simulink model "VaRedoxFlowBattery"  (R2025b)
settings: Solver=daessc  StartTime=0.0  StopTime=217080  FixedStep=1  MaxStep=1  RelTol=1e-3
libraries: fl_lib x4, nesl_utility x2, energyStorage_lib x1
settings Model: Creator=The MathWorks, Inc.  LastModifiedBy=skota
settings DataIOCC: ReturnWorkspaceOutputs=off
settings RTWCC: GPUComputeCapability=3.5
settings SimscapeCC: SimscapeLogType=all  SimscapeLogName=simlog_vrfbResults  SimscapeLogLimitData=off

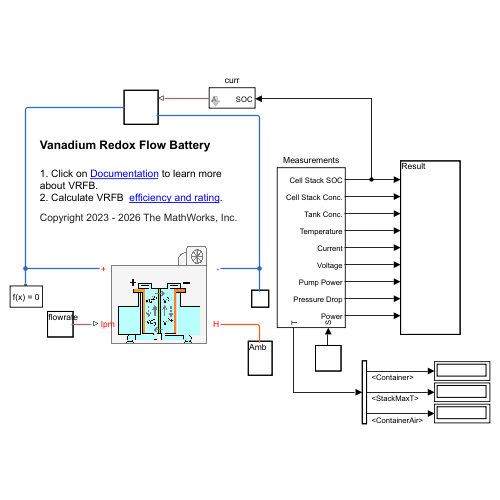
[thumbnail: Simulink's stored preview of the top-level diagram]
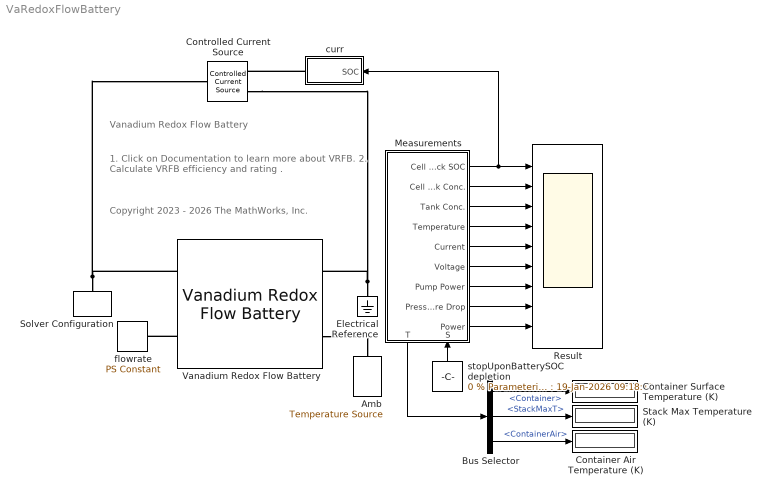
== system VaRedoxFlowBattery ==
  note: Copyright 2023 - 2026 The MathWorks, Inc.
  note: Vanadium Redox Flow Battery
  note: 1. Click on Documentation to learn more about VRFB.
      | 2. Calculate VRFB efficiency and rating .
  Amb : fl_lib/Thermal/Thermal Sources/Temperature Source  temperature=280 K
  Bus Selector : BusSelector  OutputSignals=Container,StackMaxT,ContainerAir
  Container Air Temperature (K) : Display
  Container Surface Temperature (K) : Display
  Controlled Current Source : fl_lib/Electrical/Electrical Sources/Controlled Current Source
  Electrical Reference : fl_lib/Electrical/Electrical Elements/Electrical Reference
  Measurements : Subsystem
      settings: PortSchema="{\"entries\":[{\"content\":{\"sides\":[{\"content\":{},\"type\":\"ConnectorPlacement.EquallySpacedRectSide\",\"uuid\":\"8b02043d-c9ac-404f-b44e-e3d149381142\"},{\"content\":{\"connectorIds\":[\"Out1\",\"Out2\",\"Out3\",\"Out4\",\"Out5\",\"Out6\",\"Out7\",\"Out8\",\"Out9\"],\"side\":\"RIGHT\"},\"type\":\"ConnectorPlacement.EquallySpacedRectSide\",\"uuid\":\"db8b3d67-eb39-4295-a851-710d35a8f7cb\"},{\"content\":{\"side\":\"TOP\"},\"type\":\"ConnectorPlacement.EquallySpacedRectSide\",\"uuid\":\"c6df1df3-7bc2-4a42-8cb6-fa58ab6e8d6e\"},{\"content\":{\"connectorIds\":[\"Out10\",\"In1\"],\"side\":\"BOTTOM\"},\"type\":\"ConnectorPlacement.EquallySpacedRectSide\",\"uuid\":\"3b6ba19c-eafa-4b58-a7a0-e301da792125\"}]},\"type\":\"ConnectorPlacement.EquallySpacedConnector\",\"uuid\":\"ea0fc1df-6747-461f-bfb1-e7381007efb8\"}],\"packageUris\":[\"http://schema.mathworks.com/mf0/Connector/R2020b\"],\"version\":\"1.0\"}"
  Result : Scope  NumInputPorts=9
      settings: ActiveDisplayYMinimum=-0.12365877298293816  ActiveDisplayYMaximum=1.1137398636647708
  Solver Configuration : nesl_utility/Solver Configuration  PhysicalDomain=network_engine_domain  SubClassName=solver  LeftPortType=input  RightPortType=generic  Tones=[]  Harmonics=[]  SimulateNoise=off  Profile=off  UseLocalSampling=off  EnableSwitchedLinearOptims=on  FrequencyDomain=off  UseCCode=off  RelTol=0.001  AbsTol=0.001  MinStep=1e-09  ToWorkspace=off  RevertToSquareIcSolve=off  NumHomotopyIterations=100  PhasorMode=off  PhasorModeNumHarmonics=1  ConsistencySolver=NEWTON_XTOL_AFTER_FTOL  CanonicalOrdering=UNORDERED  OptimizeIntermediates=UNOPTIMIZED  IndexReductionMethod=DerivativeReplacement  DoDC=off  ResidualTolerance=1e-09  ConsistencyTolSource=GLOBAL  ConsistencyAbsTol=0.001  ConsistencyRelTol=0.001  ConsistencyTolFactor=0.001  UseLocalSolver=off  LocalSolverChoice=NE_BACKWARD_EULER_ADVANCER  ResolveIndetEquations=on  FunctionEvalNumThread=1  LocalSolverSampleTime=0.01  DoFixedCost=off  MaxNonlinIter=10  MaxModeIter=2  ComputeImpulses=off  ImpulseIterations=2  LinearAlgebra=auto  LinearAlgebraNumThread=0  EquationFormulation=NE_TIME_EF  DelaysMemoryBudget=1024  AutomaticFiltering=on  FilteringTimeConstant=0.001  PartitionStorageMethod=AS_NEEDED  PartitionMemoryBudget=1024  PartitionMethod=ROBUST  MultibodyUseLocalSolver=off  MultibodyLocalSolverChoice=ODE1  MultibodyLocalSolverSampleTime=0.001
  Stack Max Temperature (K) : Display
  Vanadium Redox Flow Battery : energyStorage_lib/Vanadium Redox Flow Battery  flowrateLUT=[5, 10, 20, 40, 80] lpm  thermalManagement=vanadiumRedoxFlowThermalModel.enabled  temperatureLUT=[293, 300, 313] K  initialTsys=280 K  SOC=0.99  electrolyteDen=1000 kg/m^3  electrolyteCp=800 J/(K*kg)  electrolyteKinVis=3.9e-6 m^2/s  crossDiffModel=vanadiumRedoxFlowChemistry.disabled  thMemb=1e-3 m  diffCoeff2=4.31e-12 m^2/s  diffCoeff3=1.92e-12 m^2/s  diffCoeff4=6.53e-12 m^2/s  diffCoeff5=3.78e-12 m^2/s  activationE=17341 W*s/mol  electrolyteK=1 1/(Ohm*m)  minStateOfCharge=1e-4  maxStateOfCharge=0.9999  msgWarn=simscape.enum.assert.action.none  molar=2 mol/l  V0=1.3 V  LUTdischgR0=0.1 * ones(3, 5) Ohm  LUTdischgRes=0.1 * ones(3, 5) Ohm  LUTdischgTau=10 * ones(3, 5) s  LUTchgR0=0.1 * ones(3, 5) Ohm  LUTchgRes=0.1 * ones(3, 5) Ohm  LUTchgTau=10 * ones(3, 5) s  stackLen=0.15 m  stackWid=0.30 m  stackHgt=0.30 m  stackMassCp=324000 J/K  stackPrDropLUT=[100, 110, 120, 130, 140] Pa  pipeLength=1 m  pipeDia=1e-2 m  pipeArea=0.01 m^2  pipeRoughness=15e-6 m  Nc=20  Ns=10  Np=2  seriesFlowMalDistr=ones(1, 10)  shuntResModel=vanadiumRedoxFlowShuntCurrModel.disabled  shuntRes=1000 Ohm  containerVolume=0.5 m^3  containerArea=10 m^2  containerThermalmass=90000 J/K  nFans=5  fanCapacity=80 m^3/hr  extHTC=20 W/(K*m^2)  F=96485 C/mol  R=8.314 J/(K*mol)  Cmin=0 mol/m^3  openSw=1e-8 1/Ohm  flUnit=1 / 60000 m^3/(lpm*s)  containerAirCp=700 J/(K*kg)  containerAirDen=1.2 kg/m^3  ReLaminar=2000  ReTurbulent=4000  darcyFriction=64  vSwitchOpen_specify=off  vSwitchOpen_priority=None  vSwitchOpen=0 V  vSwitchOpen_nominal_specify=off  vSwitchOpen_nominal_value=1  vSwitchOpen_nominal_unit=V  portH_specify=off  portH_priority=None  portH=0 W  portH_nominal_specify=off  portH_nominal_value=1  portH_nominal_unit=W  tankNegT_specify=off  tankNegT_priority=High  tankNegT=298 K  tankNegT_nominal_specify=off  tankNegT_nominal_value=1  tankNegT_nominal_unit=K  tankPosT_specify=off  tankPosT_priority=High  tankPosT=298 K  tankPosT_nominal_specify=off  tankPosT_nominal_value=1  tankPosT_nominal_unit=K  i_specify=off  i_priority=None  i=0 A  i_nominal_specify=off  i_nominal_value=1  i_nominal_unit=A  is_specify=off  is_priority=None  is=0 A  is_nominal_specify=off  is_nominal_value=1  is_nominal_unit=A  systemPrDrop_specify=off  systemPrDrop_priority=None  systemPrDrop=0 Pa  systemPrDrop_nominal_specify=off  systemPrDrop_nominal_value=1  systemPrDrop_nominal_unit=Pa  shuntCurrPercent_specify=off  shuntCurrPercent_priority=None  shuntCurrPercent=0  shuntCurrPercent_nominal_specify=off  shuntCurrPercent_nominal_value=1  shuntCurrPercent_nominal_unit=1
  curr : Subsystem  mask{minSOC=1e-4, maxSOC=0.9999, initialSOC=0.99 % Parameterized on : 19-Jan-2026 09:17:42, current=-30 % Parameterized on : 19-Jan-2026 09:17:42}
      mask prompts: minSOC "Minimum SOC"; maxSOC "Maximum SOC"; initialSOC "Initial SOC"; current "Current (A)"
      settings: PortSchema="{\"entries\":[{\"content\":{\"sides\":[{\"content\":{\"connectorIds\":[\"LConn1\"]},\"type\":\"ConnectorPlacement.EquallySpacedRectSide\",\"uuid\":\"8f065474-aca1-43fd-818c-991450ade969\"},{\"content\":{\"connectorIds\":[\"In1\"],\"side\":\"RIGHT\"},\"type\":\"ConnectorPlacement.EquallySpacedRectSide\",\"uuid\":\"8684384d-eee1-4ef9-8ccb-1008bfac02ea\"},{\"content\":{\"side\":\"TOP\"},\"type\":\"ConnectorPlacement.EquallySpacedRectSide\",\"uuid\":\"24e81199-7765-4e7a-8bd0-061ca1263c91\"}]},\"type\":\"ConnectorPlacement.EquallySpacedConnector\",\"uuid\":\"937b71f9-e393-4054-814d-f0ac9beb7810\"}],\"packageUris\":[\"http://schema.mathworks.com/mf0/Connector/R2020b\"],\"version\":\"1.0\"}"
  flowrate : fl_lib/Physical Signals/Sources/PS Constant  constant=20 % Parameterized on : 19-Jan-2026 09:17:08 m^3/hr
  stopUponBatterySOCdepletion : Constant  Value=0 % Parameterized on : 19-Jan-2026 09:18:15
  wires:
  Measurements/1(Cell Stack SOC) -> curr/1(SOC), Result/1
  Measurements/2(Cell Stack Conc.) -> Result/2
  Measurements/3(Tank Conc.) -> Result/3
  Measurements/4(Temperature) -> Result/4
  Measurements/5(Current) -> Result/5
  Measurements/6(Voltage) -> Result/6
  Measurements/7(Pump Power) -> Result/7
  Measurements/8(Pressure Drop) -> Result/8
  Measurements/9(Power) -> Result/9
  stopUponBatterySOCdepletion/1 -> Measurements/1(S)
  Measurements/10(T) -> Bus Selector/1
  Bus Selector/1 -> Container Surface Temperature (K)/1  "<Container>"
  Bus Selector/2 -> Stack Max Temperature (K)/1  "<StackMaxT>"
  Bus Selector/3 -> Container Air Temperature (K)/1  "<ContainerAir>"
  connections:
  Electrical Reference/LConn1 -- Vanadium Redox Flow Battery/RConn1 -- Controlled Current Source/RConn2
  Solver Configuration/RConn1 -- Vanadium Redox Flow Battery/LConn1 -- Controlled Current Source/LConn1
  Vanadium Redox Flow Battery/LConn2 -- flowrate/RConn1
  curr/LConn1 -- Controlled Current Source/RConn1
  Vanadium Redox Flow Battery/RConn2 -- Amb/LConn1

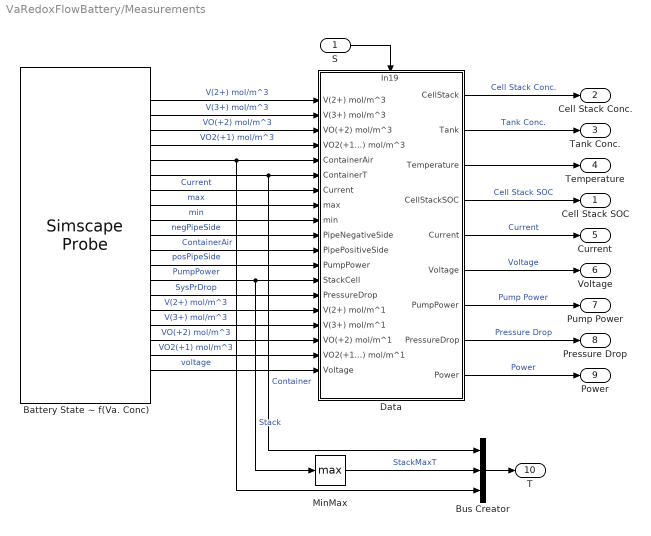
== system VaRedoxFlowBattery/Measurements ==
  S : Inport
  Battery State ~ f(Va. Conc) : SimscapeProbe  BoundBlock=464  Variables="{\"cellC2vec\":{\"Probing\":\"ON\"},\"cellC3vec\":{\"Probing\":\"ON\"},\"cellC4vec\":{\"Probing\":\"ON\"},\"cellC5vec\":{\"Probing\":\"ON\"},\"containerAirT\":{\"Probing\":\"ON\"},\"containerT\":{\"Probing\":\"ON\"},\"i\":{\"Probing\":\"ON\"},\"maxCellStackSOC\":{\"Probing\":\"ON\"},\"minCellStackSOC\":{\"Probing\":\"ON\"},\"pipeNegSideT\":{\"Probing\":\"ON\"},\"pipePosSideT\":{\"Probing\":\"ON\"},\"pump_power\":{\"Probing\":\"ON\"},\"stackCellT\":{\"Probing\":\"ON\"},\"stateOfCharge\":{\"Probing\":\"OFF\"},\"systemPrDrop\":{\"Probing\":\"ON\"},\"tankC2\":{\"Probing\":\"ON\"},\"tankC3\":{\"Probing\":\"ON\"},\"tankC4\":{\"Probing\":\"ON\"},\"tankC5\":{\"Probing\":\"ON\"},\"v\":{\"Probing\":\"ON\"}}"
  Bus Creator : BusCreator  Inputs=3
  Data : Subsystem
      settings: PortSchema="{\"entries\":[{\"content\":{\"sides\":[{\"content\":{\"connectorIds\":[\"In1\",\"In2\",\"In3\",\"In4\",\"In5\",\"In6\",\"In7\",\"In8\",\"In9\",\"In10\",\"In11\",\"In12\",\"In13\",\"In14\",\"In15\",\"In16\",\"In17\",\"In18\",\"In19\"]},\"type\":\"ConnectorPlacement.EquallySpacedRectSide\",\"uuid\":\"59facf9b-f4b6-4a75-b324-a88668e355b1\"},{\"content\":{\"connectorIds\":[\"Out1\",\"Out2\",\"Out3\",\"Out4\",\"Out5\",\"Out6\",\"Out7\",\"Out8\",\"Out9\"],\"side\":\"RIGHT\"},\"type\":\"ConnectorPlacement.EquallySpacedRectSide\",\"uuid\":\"b0c5b6f3-807f-48fc-b27f-80d0cc8639cc\"},{\"content\":{\"connectorIds\":[\"In20\"],\"side\":\"TOP\"},\"type\":\"ConnectorPlacement.EquallySpacedRectSide\",\"uuid\":\"469f6e69-9243-476d-8eba-60bb5b8ef42c\"}]},\"type\":\"ConnectorPlacement.EquallySpacedConnector\",\"uuid\":\"25ec820e-cccc-4d37-921c-f8b16cbf06a5\"}],\"packageUris\":[\"http://schema.mathworks.com/mf0/Connector/R2020b\"],\"version\":\"1.0\"}"
  MinMax : MinMax  Function=max
  Cell Stack SOC : Outport
  Cell Stack Conc. : Outport  Port=2
  Tank Conc. : Outport  Port=3
  Temperature : Outport  Port=4
  Current : Outport  Port=5
  Voltage : Outport  Port=6
  Pump Power : Outport  Port=7
  Pressure Drop : Outport  Port=8
  Power : Outport  Port=9
  T : Outport  Port=10
  wires:
  Data/1(CellStack) -> Cell Stack Conc./1  "Cell Stack Conc."
  Battery State ~ f(Va. Conc)/15 -> Data/15(V(2+) mol/m^1)  "V(2+) mol/m^3"
  Data/2(Tank) -> Tank Conc./1  "Tank Conc."
  Battery State ~ f(Va. Conc)/5 -> Bus Creator/3, Data/5(ContainerAir)  "ContainerAir"
  Battery State ~ f(Va. Conc)/10 -> Data/10(PipeNegativeSide)  "negPipeSide"
  Battery State ~ f(Va. Conc)/9 -> Data/9(min)  "min"
  Data/4(CellStackSOC) -> Cell Stack SOC/1  "Cell Stack SOC"
  Battery State ~ f(Va. Conc)/17 -> Data/17(VO(+2) mol/m^1)  "VO(+2) mol/m^3"
  S/1 -> Data/20(In19)
  Battery State ~ f(Va. Conc)/13 -> MinMax/1, Data/13(StackCell)  "Stack"
  Battery State ~ f(Va. Conc)/3 -> Data/3(VO(+2) mol/m^3)  "VO(+2) mol/m^3"
  Data/6("Voltage ") -> Voltage/1  "Voltage"
  Battery State ~ f(Va. Conc)/7 -> Data/7(Current)  "Current"
  Data/8("PressureDrop ") -> Pressure Drop/1  "Pressure Drop"
  Data/3(Temperature) -> Temperature/1
  Battery State ~ f(Va. Conc)/4 -> Data/4(VO2(+1) mol/m^3)  "VO2(+1) mol/m^3"
  Battery State ~ f(Va. Conc)/16 -> Data/16(V(3+) mol/m^1)  "V(3+) mol/m^3"
  Battery State ~ f(Va. Conc)/18 -> Data/18(VO2(+1) mol/m^1)  "VO2(+1) mol/m^3"
  Data/7("PumpPower ") -> Pump Power/1  "Pump Power"
  Data/5("Current ") -> Current/1  "Current"
  Battery State ~ f(Va. Conc)/1 -> Data/1(V(2+) mol/m^3)  "V(2+) mol/m^3"
  Battery State ~ f(Va. Conc)/8 -> Data/8(max)  "max"
  Battery State ~ f(Va. Conc)/6 -> Bus Creator/1, Data/6(ContainerT)  "Container"
  Battery State ~ f(Va. Conc)/11 -> Data/11(PipePositiveSide)  "posPipeSide"
  Battery State ~ f(Va. Conc)/12 -> Data/12(PumpPower)  "PumpPower"
  Battery State ~ f(Va. Conc)/14 -> Data/14(PressureDrop)  "SysPrDrop"
  Battery State ~ f(Va. Conc)/2 -> Data/2(V(3+) mol/m^3)  "V(3+) mol/m^3"
  Data/9(Power) -> Power/1  "Power"
  MinMax/1 -> Bus Creator/2  "StackMaxT"
  Bus Creator/1 -> T/1
  Battery State ~ f(Va. Conc)/19 -> Data/19(Voltage)  "voltage"

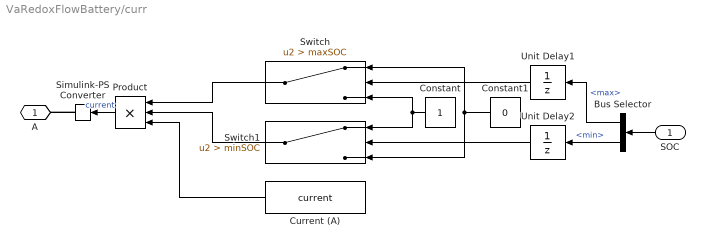
== system VaRedoxFlowBattery/curr ==
  SOC : Inport
  Bus Selector : BusSelector  OutputSignals=max,min
  Constant : Constant
  Constant1 : Constant  Value=0
  Current (A) : Constant  Value=current
  Product : Product  Inputs=3
  Simulink-PS Converter : nesl_utility/Simulink-PS Converter  PhysicalDomain=network_engine_domain  SubClassName=ps_input  LeftPortType=input  RightPortType=output  PseudoPeriodic=off  Frequencies=[]  NoiseDistribution=none  NoiseParameters=[]  Unit=A  AffineConversion=off  FilteringAndDerivatives=filter  SimscapeFilterOrder=1  InputFilterTimeConstant=0.001  UdotUserProvided=0
  Switch : Switch  Criteria=u2 > Threshold  Threshold=maxSOC  SaturateOnIntegerOverflow=off  InputSameDT=off
  Switch1 : Switch  Criteria=u2 > Threshold  Threshold=minSOC  SaturateOnIntegerOverflow=off  InputSameDT=off
  Unit Delay1 : UnitDelay  InitialCondition=initialSOC  SampleTime=-1
  Unit Delay2 : UnitDelay  InitialCondition=initialSOC  SampleTime=-1
  "A " : PMIOPort  Side=Left
  wires:
  Current (A)/1 -> Product/3
  Switch1/1 -> Product/2
  Switch/1 -> Product/1
  Bus Selector/2 -> Unit Delay2/1  "<min>"
  Constant1/1 -> Switch/1, Switch1/3
  Product/1 -> Simulink-PS Converter/1  "current"
  Constant/1 -> Switch/3, Switch1/1
  SOC/1 -> Bus Selector/1
  Unit Delay1/1 -> Switch/2
  Unit Delay2/1 -> Switch1/2
  Bus Selector/1 -> Unit Delay1/1  "<max>"
  connections:
  Simulink-PS Converter/RConn1 -- "A "/RConn1

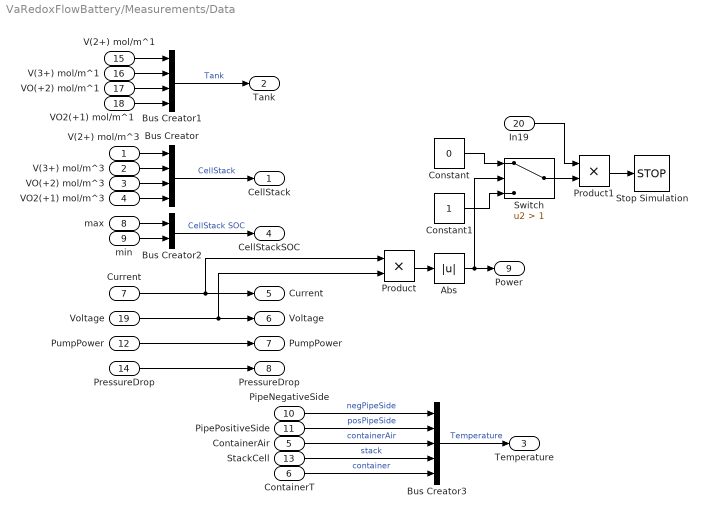
== system VaRedoxFlowBattery/Measurements/Data ==
  V(2+) mol/m^3 : Inport
  V(3+) mol/m^3 : Inport  Port=2
  VO(+2) mol/m^3 : Inport  Port=3
  VO2(+1) mol/m^3 : Inport  Port=4
  ContainerAir : Inport  Port=5
  ContainerT : Inport  Port=6
  Current : Inport  Port=7
  max : Inport  Port=8
  min : Inport  Port=9
  PipeNegativeSide : Inport  Port=10
  PipePositiveSide : Inport  Port=11
  PumpPower : Inport  Port=12
  StackCell : Inport  Port=13
  PressureDrop : Inport  Port=14
  V(2+) mol/m^1 : Inport  Port=15
  V(3+) mol/m^1 : Inport  Port=16
  VO(+2) mol/m^1 : Inport  Port=17
  VO2(+1) mol/m^1 : Inport  Port=18
  Voltage : Inport  Port=19
  In19 : Inport  Port=20
  Abs : Abs  SaturateOnIntegerOverflow=off
  Bus Creator : BusCreator  Inputs=4
  Bus Creator1 : BusCreator  Inputs=4
  Bus Creator2 : BusCreator  Inputs=2
  Bus Creator3 : BusCreator  Inputs=5
  Constant : Constant  Value=0
  Constant1 : Constant
  Product : Product
  Product1 : Product
  Stop Simulation : Stop
  Switch : Switch  Criteria=u2 > Threshold  Threshold=1  SaturateOnIntegerOverflow=off  InputSameDT=off
  CellStack : Outport
  Tank : Outport  Port=2
  Temperature : Outport  Port=3
  CellStackSOC : Outport  Port=4
  "Current " : Outport  Port=5
  "Voltage " : Outport  Port=6
  "PumpPower " : Outport  Port=7
  "PressureDrop " : Outport  Port=8
  Power : Outport  Port=9
  wires:
  max/1 -> Bus Creator2/1
  V(2+) mol/m^1/1 -> Bus Creator1/1
  PipeNegativeSide/1 -> Bus Creator3/1  "negPipeSide"
  min/1 -> Bus Creator2/2
  VO(+2) mol/m^1/1 -> Bus Creator1/3
  VO2(+1) mol/m^1/1 -> Bus Creator1/4
  V(3+) mol/m^3/1 -> Bus Creator/2
  ContainerAir/1 -> Bus Creator3/3  "containerAir"
  V(2+) mol/m^3/1 -> Bus Creator/1
  StackCell/1 -> Bus Creator3/4  "stack"
  VO(+2) mol/m^3/1 -> Bus Creator/3
  V(3+) mol/m^1/1 -> Bus Creator1/2
  VO2(+1) mol/m^3/1 -> Bus Creator/4
  PipePositiveSide/1 -> Bus Creator3/2  "posPipeSide"
  Bus Creator/1 -> CellStack/1  "CellStack"
  Bus Creator3/1 -> Temperature/1  "Temperature"
  Bus Creator2/1 -> CellStackSOC/1  "CellStack SOC"
  Current/1 -> Product/1, "Current "/1
  Voltage/1 -> Product/2, "Voltage "/1
  PressureDrop/1 -> "PressureDrop "/1
  PumpPower/1 -> "PumpPower "/1
  Bus Creator1/1 -> Tank/1  "Tank"
  Product/1 -> Abs/1
  Abs/1 -> Switch/2, Power/1
  Constant/1 -> Switch/1
  Constant1/1 -> Switch/3
  Switch/1 -> Product1/2
  Product1/1 -> Stop Simulation/1
  In19/1 -> Product1/1
  ContainerT/1 -> Bus Creator3/5  "container"
